simulink model "processSim"  (R2017b)
settings: Solver=VariableStepAuto  StartTime=0.0  StopTime=20  RelTol=1e-3
libraries: hdlsllib x7, dspsrcs4 x1
settings Model: Creator=pc  LastModifiedBy=pc
settings DataIOCC: LimitDataPoints=on  SaveOutput=off  SaveTime=off
settings OptimizationCC: BlockReduction=off  BooleanDataType=off  LifeSpan=inf
settings DebuggingCC: SaveWithParameterizedLinksMsg=none  UnderspecifiedInitializationDetection=Classic  MergeDetectMultiDrivingBlocksExec=none  SignalResolutionControl=TryResolveAllWithWarning  AllowSymbolicDim=off  SFUnexpectedBacktrackingDiag=warning  SFNoUnconditionalDefaultTransitionDiag=warning  SFExecutionAtInitializationDiag=none
settings HardwareCC: TargetUnknown=on
settings CodeAppCC: StateflowObjectComments=on
settings GRTTargetCC: TargetLangStandard=C89/C90 (ANSI)  GeneratePreprocessorConditionals=Disable all

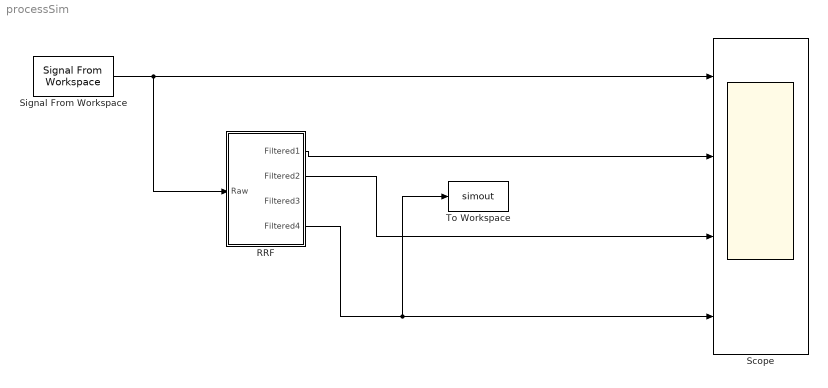
== system processSim ==
  RRF : Subsystem
  Scope : Scope  NumInputPorts=4
  Signal From Workspace : dspsrcs4/Signal From Workspace  X=fix_noiseECG  Ts=1/250  nsamps=1  OutputAfterFinalValue=Setting to zero  ignoreOrWarnInputAndFrameLengths=off  OutputFrames=off
  To Workspace : ToWorkspace  VariableName=simout  SampleTime=-1
      settings: Save2DSignal=2-D array (concatenate along first dimension)
  wires:
  Signal From Workspace/1 -> RRF/1("Raw "), Scope/1
  RRF/1(Filtered1) -> Scope/2
  RRF/2(Filtered2) -> Scope/3
  RRF/4(Filtered4) -> To Workspace/1, Scope/4

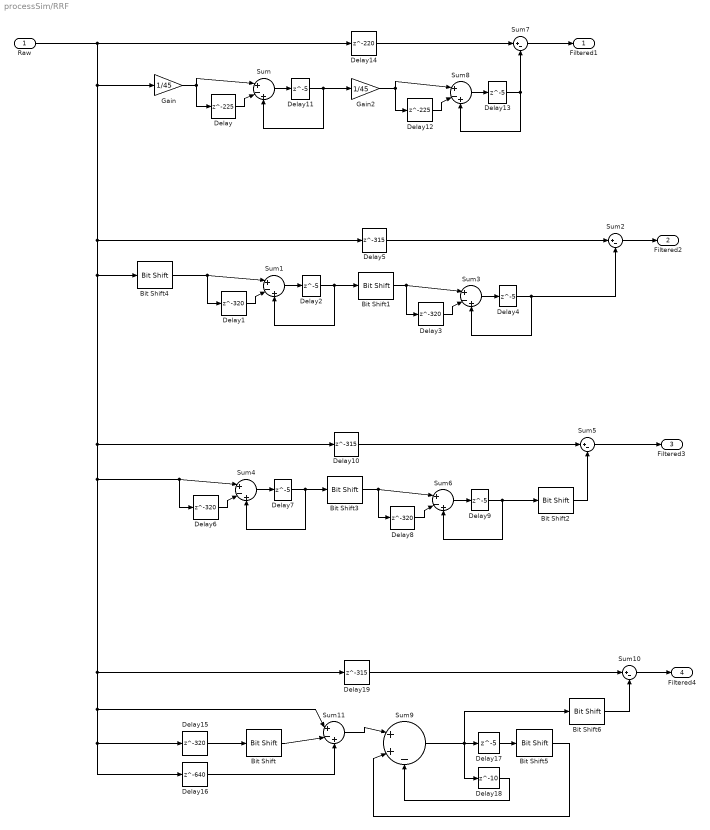
== system processSim/RRF ==
  "Raw " : Inport
  Bit Shift : hdlsllib/Logic and Bit Operations/Bit Shift  mode=Shift Left Logical  N=1
      settings: SourceProductName=HDL Coder  SourceProductBaseCode=HD
  Bit Shift{1..4} (4 alike) : hdlsllib/Logic and Bit Operations/Bit Shift  mode=Shift Right Arithmetic  N=6
      settings: SourceProductName=HDL Coder  SourceProductBaseCode=HD
  Bit Shift5 : hdlsllib/Logic and Bit Operations/Bit Shift  mode=Shift Left Logical  N=1
      settings: SourceProductName=HDL Coder  SourceProductBaseCode=HD
  Bit Shift6 : hdlsllib/Logic and Bit Operations/Bit Shift  mode=Shift Right Arithmetic  N=12
      settings: SourceProductName=HDL Coder  SourceProductBaseCode=HD
  Delay : Delay  DelayLength=225  InitialCondition=0
  Delay{1,3,6,8,15} (5 alike) : Delay  DelayLength=320  InitialCondition=0
  Delay10 : Delay  DelayLength=315  InitialCondition=0
  Delay{2,4,7,9,11,13,17} (7 alike) : Delay  DelayLength=5  InitialCondition=0
  Delay12 : Delay  DelayLength=225  InitialCondition=0
  Delay14 : Delay  DelayLength=220  InitialCondition=0
  Delay16 : Delay  DelayLength=640  InitialCondition=0
  Delay18 : Delay  DelayLength=10  InitialCondition=0
  Delay19 : Delay  DelayLength=315  InitialCondition=0
  Delay5 : Delay  DelayLength=315  InitialCondition=0
  Gain : Gain  Gain=1/45  OutDataTypeStr=int32
  Gain2 : Gain  Gain=1/45  OutDataTypeStr=int32
  Sum{,1,3..4,6,8,11} (7 alike) : Sum  Inputs=|+-+
  Sum{2,5,7,10} (4 alike) : Sum  Inputs=|+-
  Sum9 : Sum  Inputs=|++-
  Filtered1 : Outport
  Filtered2 : Outport  Port=2
  Filtered3 : Outport  Port=3
  Filtered4 : Outport  Port=4
  wires:
  Delay13/1 -> Sum7/2, Sum8/3
  Sum8/1 -> Delay13/1
  Delay14/1 -> Sum7/1
  Delay11/1 -> Gain2/1, Sum/3
  Delay12/1 -> Sum8/2
  Sum/1 -> Delay11/1
  Gain2/1 -> Delay12/1, Sum8/1
  Delay/1 -> Sum/2
  Gain/1 -> Delay/1, Sum/1
  Sum7/1 -> Filtered1/1
  Bit Shift4/1 -> Delay1/1, Sum1/1
  Delay1/1 -> Sum1/2
  Bit Shift1/1 -> Delay3/1, Sum3/1
  Sum1/1 -> Delay2/1
  Delay2/1 -> Bit Shift1/1, Sum1/3
  Delay3/1 -> Sum3/2
  Sum2/1 -> Filtered2/1
  Delay4/1 -> Sum2/2, Sum3/3
  Delay5/1 -> Sum2/1
  Sum3/1 -> Delay4/1
  Delay7/1 -> Bit Shift3/1, Sum4/3
  Delay8/1 -> Sum6/2
  Sum4/1 -> Delay7/1
  Delay6/1 -> Sum4/2
  Sum6/1 -> Delay9/1
  Delay10/1 -> Sum5/1
  Delay9/1 -> Bit Shift2/1, Sum6/3
  Bit Shift2/1 -> Sum5/2
  Bit Shift3/1 -> Delay8/1, Sum6/1
  Sum5/1 -> Filtered3/1
  Delay16/1 -> Sum11/3
  Sum9/1 -> Bit Shift6/1, Delay18/1, Delay17/1
  Delay18/1 -> Sum9/3
  Bit Shift5/1 -> Sum9/2
  Delay19/1 -> Sum10/1
  Sum11/1 -> Sum9/1
  Delay17/1 -> Bit Shift5/1
  Delay15/1 -> Bit Shift/1
  Bit Shift/1 -> Sum11/2
  "Raw "/1 -> Sum11/1, Delay15/1, Delay16/1, Delay19/1, Delay6/1, Sum4/1, Delay10/1, Bit Shift4/1, Delay5/1, Gain/1, Delay14/1
  Sum10/1 -> Filtered4/1
  Bit Shift6/1 -> Sum10/2
